simulink model "Formation_Controller"  (R2022b)
settings: Solver=FixedStepDiscrete  StartTime=0.0  StopTime=10.0  FixedStep=CTRL_CONST.dt  RelTol=1e-3
undefined symbols (not defined in the file or in its folder): CTRL_PARAM
libraries: simulink x1
settings Model: Creator=19114  LastModifiedBy=19114
settings OptimizationCC: DefaultParameterBehavior=Inlined  EnhancedBackFolding=on  PassReuseOutputArgsAs=Individual arguments  ZeroExternalMemoryAtStartup=off  ZeroInternalMemoryAtStartup=off  OptimizeBlockOrder=speed  DifferentSizesBufferReuse=on  OptimizationCustomize=off  EfficientTunableParamExpr=on
settings DebuggingCC: ParameterTunabilityLossMsg=error
settings SFSimCC: MATLABDynamicMemAlloc=off
settings RTWCC: Description=Embedded Coder  SystemTargetFile=ert.tlc  TemplateMakefile=ert_default_tmf
settings CodeAppCC: ForceParamTrailComments=on  IgnoreCustomStorageClasses=off  OperatorAnnotations=on  SimulinkDataObjDesc=on  SFDataObjDesc=on  InsertBlockDesc=on
settings ERTTargetCC: TargetLangStandard=C99 (ISO)  GenerateSampleERTMain=on  SupportVariableSizeSignals=on  InlinedParameterPlacement=NonHierarchical  ERTCustomFileTemplate=example_file_process.tlc

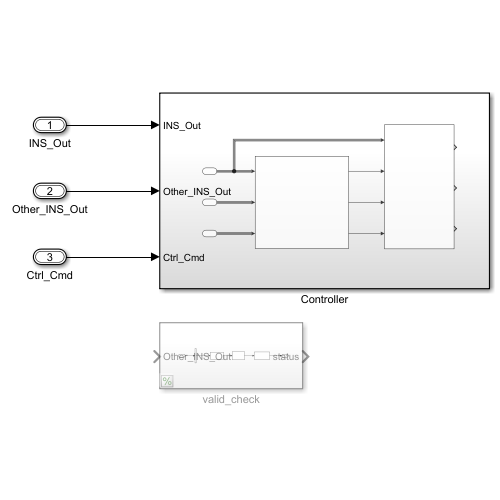
[thumbnail: Simulink's stored preview of the top-level diagram]
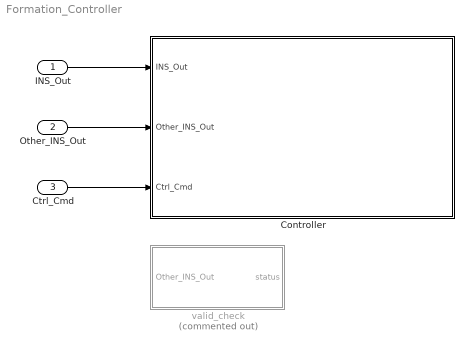
== system Formation_Controller ==
  INS_Out : Inport  OutDataTypeStr=Bus: INS_Out_Bus
  Other_INS_Out : Inport  Port=2  OutDataTypeStr=Bus: Other_INS_Out_Bus
  Ctrl_Cmd : Inport  Port=3  OutDataTypeStr=Bus: Ctrl_Cmd_Bus
  Controller : Subsystem
  valid_check : Subsystem  Commented=on
  wires:
  INS_Out/1 -> Controller/1(INS_Out)
  Other_INS_Out/1 -> Controller/2(Other_INS_Out)
  Ctrl_Cmd/1 -> Controller/3(Ctrl_Cmd)

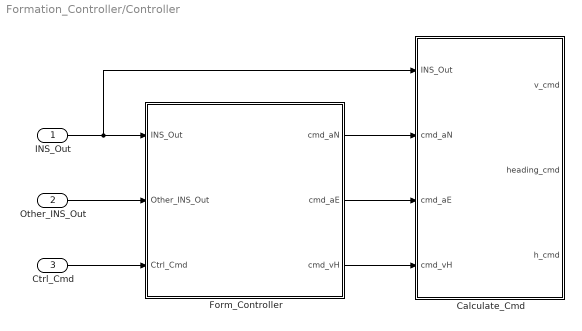
== system Formation_Controller/Controller ==
  INS_Out : Inport
  Other_INS_Out : Inport  Port=2
  Ctrl_Cmd : Inport  Port=3
  Calculate_Cmd : Subsystem
  Form_Controller : Subsystem
  wires:
  Ctrl_Cmd/1 -> Form_Controller/3(Ctrl_Cmd)
  Other_INS_Out/1 -> Form_Controller/2(Other_INS_Out)
  INS_Out/1 -> Calculate_Cmd/1(INS_Out), Form_Controller/1(INS_Out)
  Form_Controller/1(cmd_aN) -> Calculate_Cmd/2(cmd_aN)
  Form_Controller/2(cmd_aE) -> Calculate_Cmd/3(cmd_aE)
  Form_Controller/3(cmd_vH) -> Calculate_Cmd/4(cmd_vH)

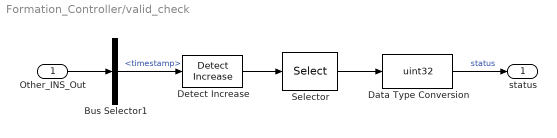
== system Formation_Controller/valid_check ==
  Other_INS_Out : Inport
  Bus Selector1 : BusSelector  OutputSignals=timestamp
  Data Type Conversion : DataTypeConversion  OutDataTypeStr=uint32  SaturateOnIntegerOverflow=off  RndMeth=Floor
  Detect Increase : simulink/Logic and Bit Operations/Detect Increase  vinit=0.0  OutDataTypeStr=boolean
  Selector : Selector  InputPortWidth=20  IndexOptions=Index vector (dialog)  Indices=[1:CTRL_PARAM.NUM_UAV]  OutputSizes=1
  status : Outport
  wires:
  Other_INS_Out/1 -> Bus Selector1/1
  Detect Increase/1 -> Selector/1
  Bus Selector1/1 -> Detect Increase/1  "<timestamp>"
  Selector/1 -> Data Type Conversion/1
  Data Type Conversion/1 -> status/1  "status"

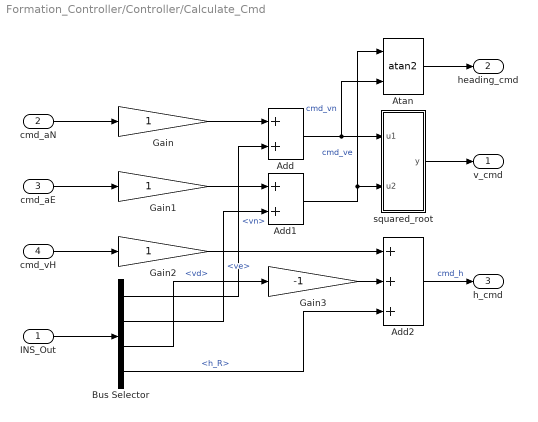
== system Formation_Controller/Controller/Calculate_Cmd ==
  INS_Out : Inport
  cmd_aN : Inport  Port=2
  cmd_aE : Inport  Port=3
  cmd_vH : Inport  Port=4
  Add : Sum
  Add1 : Sum
  Add2 : Sum  Inputs=+++
  Atan : Trigonometry  Operator=atan2
  Bus Selector : BusSelector  OutputSignals=vn,ve,vd,h_R
  Gain : Gain
  Gain1 : Gain
  Gain2 : Gain
  Gain3 : Gain  Gain=-1
  squared_root : MATLAB Function  TreatAsAtomicUnit=on
  v_cmd : Outport
  heading_cmd : Outport  Port=2
  h_cmd : Outport  Port=3
  wires:
  Bus Selector/4 -> Add2/3  "<h_R>"
  Gain3/1 -> Add2/2
  Bus Selector/3 -> Gain3/1  "<vd>"
  Gain/1 -> Add/1
  Bus Selector/1 -> Add/2  "<vn>"
  Gain1/1 -> Add1/1
  Add2/1 -> h_cmd/1  "cmd_h"
  Bus Selector/2 -> Add1/2  "<ve>"
  Gain2/1 -> Add2/1
  Add/1 -> Atan/2, squared_root/1(u1)  "cmd_vn"
  cmd_aE/1 -> Gain1/1
  cmd_vH/1 -> Gain2/1
  INS_Out/1 -> Bus Selector/1
  Add1/1 -> squared_root/2(u2), Atan/1  "cmd_ve"
  cmd_aN/1 -> Gain/1
  squared_root/1(y) -> v_cmd/1
  Atan/1 -> heading_cmd/1

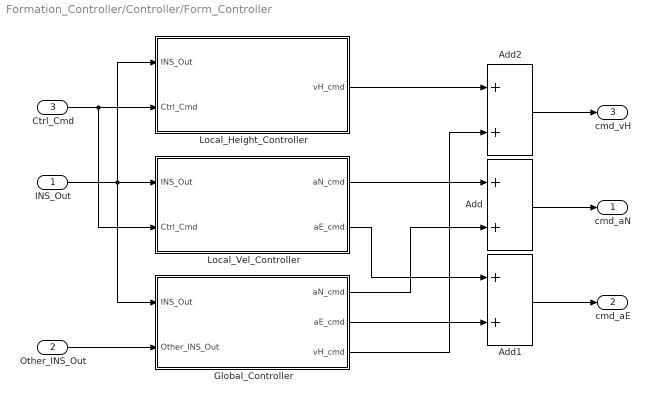
== system Formation_Controller/Controller/Form_Controller ==
  INS_Out : Inport
  Other_INS_Out : Inport  Port=2
  Ctrl_Cmd : Inport  Port=3
  Add : Sum
  Add1 : Sum
  Add2 : Sum
  Global_Controller : MATLAB Function  TreatAsAtomicUnit=on  mask{uav_id=CTRL_PARAM.UAV_ID, adj_matrix=CTRL_PARAM.ADJ_MARTIX, rel_x=CTRL_PARAM.REL_X_MATRIX, rel_y=CTRL_PARAM.REL_Y_MATRIX, rel_z=CTRL_PARAM.REL_Z_MATRIX}
      mask prompts: uav_id "uav_id (From 1)"
  Local_Height_Controller : Subsystem
  Local_Vel_Controller : Subsystem
  cmd_aN : Outport
  cmd_aE : Outport  Port=2
  cmd_vH : Outport  Port=3
  wires:
  Add/1 -> cmd_aN/1
  INS_Out/1 -> Local_Height_Controller/1(INS_Out), Global_Controller/1(INS_Out), Local_Vel_Controller/1(INS_Out)
  Ctrl_Cmd/1 -> Local_Vel_Controller/2(Ctrl_Cmd), Local_Height_Controller/2(Ctrl_Cmd)
  Local_Vel_Controller/1(aN_cmd) -> Add/1
  Other_INS_Out/1 -> Global_Controller/2(Other_INS_Out)
  Global_Controller/1(aN_cmd) -> Add/2
  Add1/1 -> cmd_aE/1
  Local_Vel_Controller/2(aE_cmd) -> Add1/1
  Local_Height_Controller/1(vH_cmd) -> Add2/1
  Global_Controller/2(aE_cmd) -> Add1/2
  Add2/1 -> cmd_vH/1
  Global_Controller/3(vH_cmd) -> Add2/2

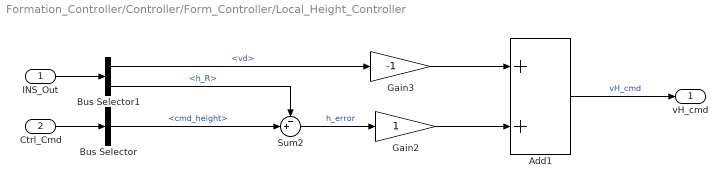
== system Formation_Controller/Controller/Form_Controller/Local_Height_Controller ==
  INS_Out : Inport
  Ctrl_Cmd : Inport  Port=2
  Add1 : Sum
  Bus Selector : BusSelector  OutputSignals=cmd_height
  Bus Selector1 : BusSelector  OutputSignals=vd,h_R
  Gain2 : Gain
  Gain3 : Gain  Gain=-1
  Sum2 : Sum  Inputs=-+|
  vH_cmd : Outport
  wires:
  Gain3/1 -> Add1/1
  Gain2/1 -> Add1/2
  INS_Out/1 -> Bus Selector1/1
  Bus Selector/1 -> Sum2/2  "<cmd_height>"
  Ctrl_Cmd/1 -> Bus Selector/1
  Bus Selector1/2 -> Sum2/1  "<h_R>"
  Sum2/1 -> Gain2/1  "h_error"
  Bus Selector1/1 -> Gain3/1  "<vd>"
  Add1/1 -> vH_cmd/1  "vH_cmd"

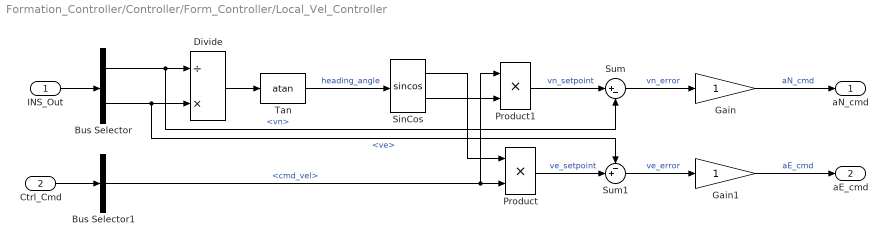
== system Formation_Controller/Controller/Form_Controller/Local_Vel_Controller ==
  INS_Out : Inport
  Ctrl_Cmd : Inport  Port=2
  Bus Selector : BusSelector  OutputSignals=vn,ve
  Bus Selector1 : BusSelector  OutputSignals=cmd_vel
  Divide : Product  Inputs=/*
  Gain : Gain
  Gain1 : Gain
  Product : Product
  Product1 : Product
  SinCos : Trigonometry  Operator=sincos
  Sum : Sum  Inputs=|+-
  Sum1 : Sum  Inputs=-+|
  Tan : Trigonometry  Operator=atan
  aN_cmd : Outport
  aE_cmd : Outport  Port=2
  wires:
  Bus Selector1/1 -> Product1/1, Product/2  "<cmd_vel>"
  Product/1 -> Sum1/2  "ve_setpoint"
  Bus Selector/2 -> Sum1/1, Divide/2  "<ve>"
  Product1/1 -> Sum/1  "vn_setpoint"
  SinCos/2 -> Product1/2
  Bus Selector/1 -> Sum/2, Divide/1  "<vn>"
  Sum1/1 -> Gain1/1  "ve_error"
  Divide/1 -> Tan/1
  Tan/1 -> SinCos/1  "heading_angle"
  SinCos/1 -> Product/1
  Sum/1 -> Gain/1  "vn_error"
  INS_Out/1 -> Bus Selector/1
  Gain1/1 -> aE_cmd/1  "aE_cmd"
  Gain/1 -> aN_cmd/1  "aN_cmd"
  Ctrl_Cmd/1 -> Bus Selector1/1

== matlab function Formation_Controller/Controller/Calculate_Cmd/squared_root ==
  data: u1 input; y output; u2 input
function y = fcn(u1, u2)

y = sqrt(u1^2 + u2^2);

== matlab function Formation_Controller/Controller/Form_Controller/Global_Controller ==
  data: INS_Out input; aN_cmd output; Other_INS_Out input; aE_cmd output; adj_matrix parameter; uav_id parameter; rel_x parameter; rel_y parameter; vH_cmd output; rel_z parameter
function [aN_cmd, aE_cmd, vH_cmd] = fcn(INS_Out, Other_INS_Out, adj_matrix, uav_id, rel_x, rel_y, rel_z)

aN_cmd = single(0);
aE_cmd = single(0);
vH_cmd = single(0);
for j = 1:size(adj_matrix, 1)
    aN_cmd = aN_cmd - adj_matrix(uav_id, j) * (INS_Out.vn - Other_INS_Out.vn(j)) + (INS_Out.x_R - Other_INS_Out.x_R(j) - rel_x(uav_id, j));
    aE_cmd = aE_cmd - adj_matrix(uav_id, j) * (INS_Out.ve - Other_INS_Out.ve(j)) + (INS_Out.y_R - Other_INS_Out.y_R(j) - rel_y(uav_id, j));
    vH_cmd = vH_cmd - adj_matrix(uav_id, j) * ((INS_Out.h_R - Other_INS_Out.h_R(j) - rel_z(uav_id, j)) + (Other_INS_Out.vd(j) - INS_Out.vd));
end
